simulink model "TST_RngMod_TrqSpdCrv"  (R2016b)
settings: Solver=FixedStepDiscrete  StartTime=0.0  StopTime=simTime  FixedStep=sampleTime  RelTol=1e-3
values from neighbouring files (symbols this model uses):
  testCase = 1    [initTST_RngMod_TrqSpdCrv_001.m]
libraries: simulink x2
settings Model: Creator=wolf072601  LastModifiedBy=wolf072601
settings DebuggingCC: SignalRangeChecking=error

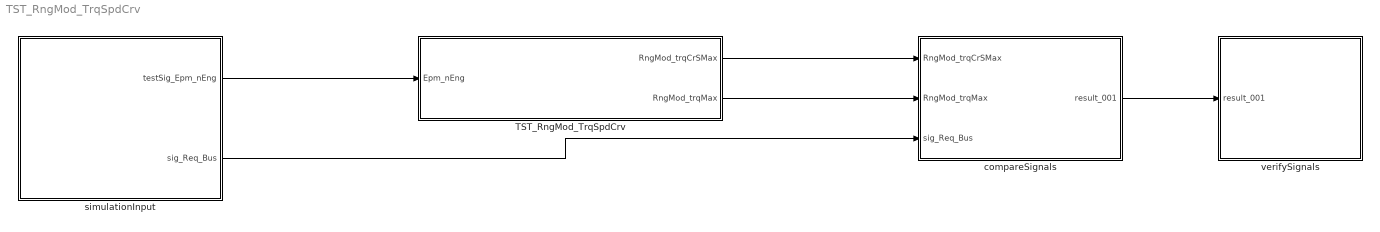
== system TST_RngMod_TrqSpdCrv ==
  TST_RngMod_TrqSpdCrv : Subsystem
  compareSignals : Subsystem
  simulationInput : Subsystem
  verifySignals : Subsystem
  wires:
  simulationInput/1(testSig_Epm_nEng) -> TST_RngMod_TrqSpdCrv/1(Epm_nEng)
  TST_RngMod_TrqSpdCrv/1(RngMod_trqCrSMax) -> compareSignals/1(RngMod_trqCrSMax)
  TST_RngMod_TrqSpdCrv/2(RngMod_trqMax) -> compareSignals/2(RngMod_trqMax)
  simulationInput/2(sig_Req_Bus) -> compareSignals/3(sig_Req_Bus)
  compareSignals/1(result_001) -> verifySignals/1(result_001)

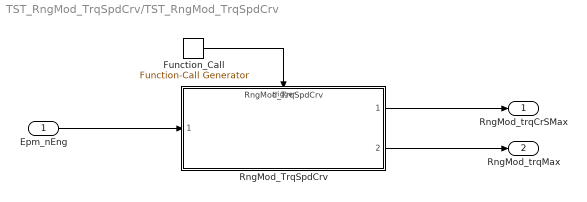
== system TST_RngMod_TrqSpdCrv/TST_RngMod_TrqSpdCrv ==
  Epm_nEng : Inport
  Function_Call : simulink/Ports & Subsystems/Function-Call Generator  sample_time=sampleTime  numberOfIterations=1
  RngMod_TrqSpdCrv : ModelReference  ModelNameDialog=RngMod_TrqSpdCrv  ModelReferenceVersion=1.2  TriggerPortName=function  TriggerPortTriggerType=function-call  TriggerPortStatesWhenEnabling=held
  RngMod_trqCrSMax : Outport
  RngMod_trqMax : Outport  Port=2
  wires:
  Function_Call/1 -> RngMod_TrqSpdCrv/Trigger
  Epm_nEng/1 -> RngMod_TrqSpdCrv/1
  RngMod_TrqSpdCrv/1 -> RngMod_trqCrSMax/1
  RngMod_TrqSpdCrv/2 -> RngMod_trqMax/1

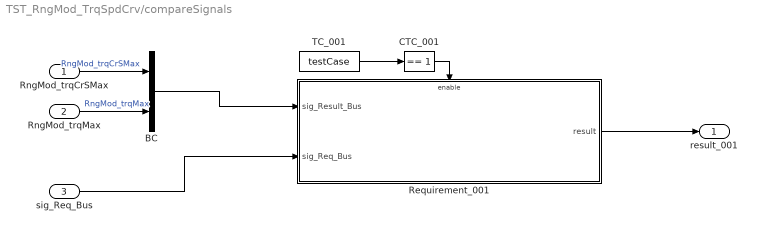
== system TST_RngMod_TrqSpdCrv/compareSignals ==
  RngMod_trqCrSMax : Inport
  RngMod_trqMax : Inport  Port=2
  sig_Req_Bus : Inport  Port=3
  BC : BusCreator  Inputs=2
  CTC_001 : simulink/Logic and Bit Operations/Compare To Constant  relop===  const=1  OutDataTypeStr=boolean
  Requirement_001 : Subsystem
  TC_001 : Constant  Value=testCase
  result_001 : Outport
  wires:
  RngMod_trqCrSMax/1 -> BC/1  "RngMod_trqCrSMax"
  RngMod_trqMax/1 -> BC/2  "RngMod_trqMax"
  TC_001/1 -> CTC_001/1
  CTC_001/1 -> Requirement_001/Enable
  sig_Req_Bus/1 -> Requirement_001/2(sig_Req_Bus)
  BC/1 -> Requirement_001/1(sig_Result_Bus)
  Requirement_001/1(result) -> result_001/1

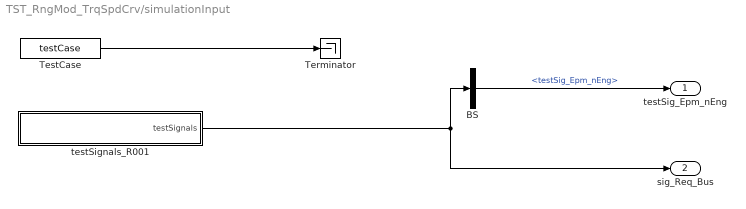
== system TST_RngMod_TrqSpdCrv/simulationInput ==
  BS : BusSelector  OutputSignals=testSig_Epm_nEng
  Terminator : Terminator
  TestCase : Constant  Value=testCase
  testSignals_R001 : Subsystem
  testSig_Epm_nEng : Outport
  sig_Req_Bus : Outport  Port=2
  wires:
  BS/1 -> testSig_Epm_nEng/1  "<testSig_Epm_nEng>"
  testSignals_R001/1(testSignals) -> BS/1, sig_Req_Bus/1
  TestCase/1 -> Terminator/1

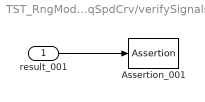
== system TST_RngMod_TrqSpdCrv/verifySignals ==
  result_001 : Inport
  Assertion_001 : Assertion  Enabled=off
  wires:
  result_001/1 -> Assertion_001/1

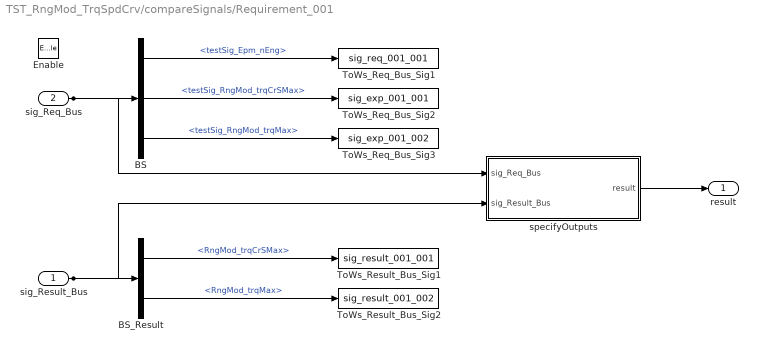
== system TST_RngMod_TrqSpdCrv/compareSignals/Requirement_001 ==
  sig_Result_Bus : Inport
  sig_Req_Bus : Inport  Port=2
  Enable : EnablePort
  BS : BusSelector  OutputSignals=testSig_Epm_nEng,testSig_RngMod_trqCrSMax,testSig_RngMod_trqMax
  BS_Result : BusSelector  OutputSignals=RngMod_trqCrSMax,RngMod_trqMax
  ToWs_Req_Bus_Sig1 : ToWorkspace  VariableName=sig_req_001_001  SaveFormat=Structure With Time
  ToWs_Req_Bus_Sig2 : ToWorkspace  VariableName=sig_exp_001_001  SaveFormat=Structure With Time
  ToWs_Req_Bus_Sig3 : ToWorkspace  VariableName=sig_exp_001_002  SaveFormat=Structure With Time
  ToWs_Result_Bus_Sig1 : ToWorkspace  VariableName=sig_result_001_001  SaveFormat=Structure With Time
  ToWs_Result_Bus_Sig2 : ToWorkspace  VariableName=sig_result_001_002  SaveFormat=Structure With Time
  specifyOutputs : Subsystem
  result : Outport
  wires:
  sig_Req_Bus/1 -> BS/1, specifyOutputs/1(sig_Req_Bus)
  BS/1 -> ToWs_Req_Bus_Sig1/1  "<testSig_Epm_nEng>"
  BS/2 -> ToWs_Req_Bus_Sig2/1  "<testSig_RngMod_trqCrSMax>"
  BS/3 -> ToWs_Req_Bus_Sig3/1  "<testSig_RngMod_trqMax>"
  sig_Result_Bus/1 -> BS_Result/1, specifyOutputs/2(sig_Result_Bus)
  BS_Result/1 -> ToWs_Result_Bus_Sig1/1  "<RngMod_trqCrSMax>"
  BS_Result/2 -> ToWs_Result_Bus_Sig2/1  "<RngMod_trqMax>"
  specifyOutputs/1(result) -> result/1

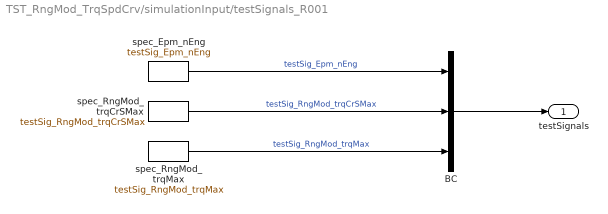
== system TST_RngMod_TrqSpdCrv/simulationInput/testSignals_R001 ==
  BC : BusCreator  Inputs=3
  spec_Epm_nEng : FromWorkspace  VariableName=testSig_Epm_nEng  Interpolate=off  OutputAfterFinalValue=Holding final value
  spec_RngMod_trqCrSMax : FromWorkspace  VariableName=testSig_RngMod_trqCrSMax  Interpolate=off  OutputAfterFinalValue=Holding final value
  spec_RngMod_trqMax : FromWorkspace  VariableName=testSig_RngMod_trqMax  Interpolate=off  OutputAfterFinalValue=Holding final value
  testSignals : Outport
  wires:
  BC/1 -> testSignals/1
  spec_Epm_nEng/1 -> BC/1  "testSig_Epm_nEng"
  spec_RngMod_trqCrSMax/1 -> BC/2  "testSig_RngMod_trqCrSMax"
  spec_RngMod_trqMax/1 -> BC/3  "testSig_RngMod_trqMax"

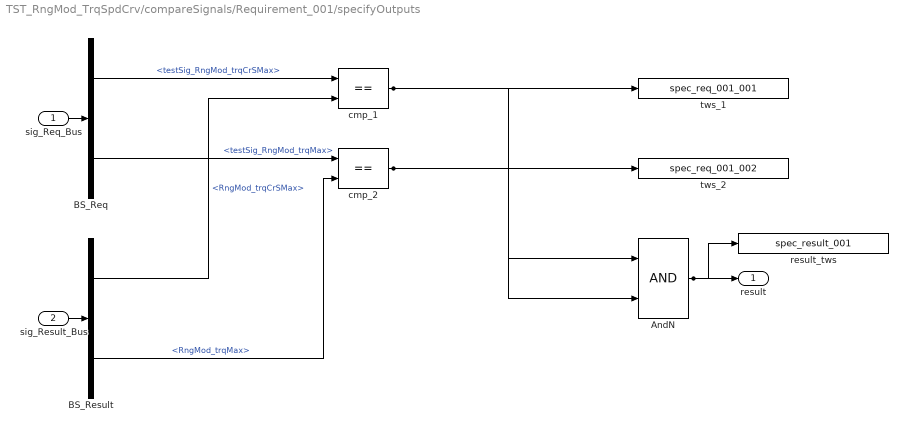
== system TST_RngMod_TrqSpdCrv/compareSignals/Requirement_001/specifyOutputs ==
  sig_Req_Bus : Inport
  sig_Result_Bus : Inport  Port=2
  AndN : Logic
  BS_Req : BusSelector  OutputSignals=testSig_RngMod_trqCrSMax,testSig_RngMod_trqMax
  BS_Result : BusSelector  OutputSignals=RngMod_trqCrSMax,RngMod_trqMax
  cmp_1 : RelationalOperator  Operator===  RndMeth=Nearest  InputSameDT=on
  cmp_2 : RelationalOperator  Operator===  RndMeth=Nearest  InputSameDT=on
  result_tws : ToWorkspace  VariableName=spec_result_001
  tws_1 : ToWorkspace  VariableName=spec_req_001_001
  tws_2 : ToWorkspace  VariableName=spec_req_001_002
  result : Outport
  wires:
  sig_Req_Bus/1 -> BS_Req/1
  sig_Result_Bus/1 -> BS_Result/1
  AndN/1 -> result/1, result_tws/1
  BS_Req/1 -> cmp_1/1  "<testSig_RngMod_trqCrSMax>"
  BS_Result/1 -> cmp_1/2  "<RngMod_trqCrSMax>"
  cmp_1/1 -> tws_1/1, AndN/1
  BS_Req/2 -> cmp_2/1  "<testSig_RngMod_trqMax>"
  BS_Result/2 -> cmp_2/2  "<RngMod_trqMax>"
  cmp_2/1 -> tws_2/1, AndN/2
